simulink model "Fx_observer"  (R2023a)
settings: Solver=ode45  StartTime=0  StopTime=25  FixedStep=0.002  RelTol=1e-3  AbsTol=1e-6
InitFcn:
  | Reff = 0.287;
  | J = 0.8;
libraries: Solver_SF x1
settings Model: ExtModeTrigMode=oneshot  Creator=ywata  LastModifiedBy=USER
settings SolverCC: AutoScaleAbsTol=off  AlgebraicLoopSolver=TrustRegion
settings DataIOCC: SaveFormat=Array  SignalLoggingSaveFormat=ModelDataLogs  ReturnWorkspaceOutputs=off  SignalLoggingName=sigsOut
settings OptimizationCC: BlockReduction=off  BooleanDataType=off  ExpressionDepthLimit=2147483647  LifeSpan=inf
settings DebuggingCC: SaveWithParameterizedLinksMsg=none  UnderspecifiedInitializationDetection=Classic  MergeDetectMultiDrivingBlocksExec=none  SignalResolutionControl=TryResolveAllWithWarning  MultiTaskDSMMsg=warning  MultiTaskCondExecSysMsg=none  FcnCallInpInsideContextMsg=warning  UnconnectedInputMsg=warning  UnconnectedOutputMsg=warning  UnconnectedLineMsg=warning  StateNameClashWarn=warning  SFUnexpectedBacktrackingDiag=warning  SFNoUnconditionalDefaultTransitionDiag=warning  SFExecutionAtInitializationDiag=none  ArithmeticOperatorsInVariantConditions=warning
settings HardwareCC: ProdBitPerPointer=32  ProdBitPerSizeT=32  ProdBitPerPtrDiffT=32  ProdLargestAtomicFloat=None  ProdIntDivRoundTo=Undefined  ProdEndianess=Unspecified  ProdWordSize=32  ProdHWDeviceType=32-bit Generic  TargetUnknown=on
settings ModelReferenceCC: PropagateSignalLabelsOutOfModel=off
settings SFSimCC: SimUseLocalCustomCode=off  CustomCodeUndefinedFunction=UseInterfaceOnly
settings RTWCC: TemplateMakefile=grt_vc.tmf  RTWUseLocalCustomCode=off
settings CodeAppCC: StateflowObjectComments=on
settings GRTTargetCC: TargetFcnLib=ansi_tfl_tmw.mat  TargetLangStandard=C89/C90 (ANSI)  CombineOutputUpdateFcns=off  GRTInterface=on
settings ConfigComp: CovMetricSettings=dw  CovSaveCumulativeToWorkspaceVar=on  CovSaveSingleToWorkspaceVar=on  CovExternalEMLEnable=off

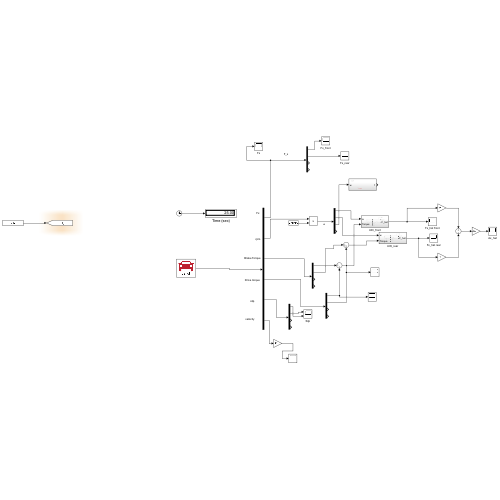
[thumbnail: Simulink's stored preview of the top-level diagram]
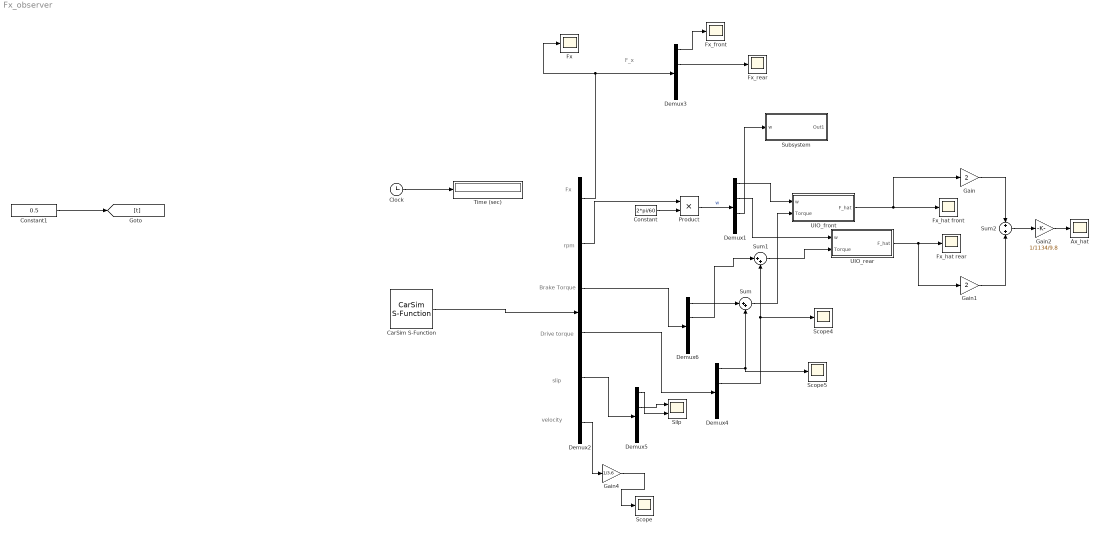
== system Fx_observer ==
  note: velocity
  note: slip
  note: Brake Torque
  note: Fx
  note: Drive torque
  note: rpm
  note: F_x
  Ax_hat : Scope
  CarSim S-Function : Solver_SF/CarSim S-Function  Priority=1  SIMFILE=simfile.sim  Run_RTs=off  vs_state_ind=Run  StopMode_ind=Vehicle Model
  Clock : Clock
  Constant : Constant  Value=2*pi/60
  Constant1 : Constant  Value=0.5
  Demux{1,3..6} (5 alike) : Demux  Outputs=[1 1 1 1]
      settings: DisplayOption=none
  Demux2 : Demux  Outputs=[4 4 4 4 4 1]
      settings: DisplayOption=none
  Fx : Scope
  Fx_front : Scope
  Fx_hat front : Scope
  Fx_hat rear : Scope
  Fx_rear : Scope
  Gain : Gain  Gain=2
  Gain1 : Gain  Gain=2
  Gain2 : Gain  Gain=1/1134/9.8
  Gain4 : Gain  Gain=1/3.6
  Product : Product
  Scope : Scope
  Scope4 : Scope
  Scope5 : Scope
  Silp : Scope  NumInputPorts=2
  Subsystem : Subsystem
  Sum : Sum  Inputs=|++
  Sum1 : Sum  Inputs=|++
  Sum2 : Sum  Inputs=+|+
  Time (sec) : Display
      settings: Format=bank  Decimation=100
  UIO_front : Subsystem
  UIO_rear : Subsystem
  wires:
  Clock/1 -> Time (sec)/1
  Demux2/1 -> Fx/1, Demux3/1
  Demux2/3 -> Demux6/1
  CarSim S-Function/1 -> Demux2/1
  Demux2/2 -> Product/1
  Constant/1 -> Product/2
  Product/1 -> Demux1/1  "w"
  Demux1/2 -> UIO_rear/1(w)
  UIO_rear/1(F_hat) -> Gain1/1, Fx_hat rear/1
  Demux3/1 -> Fx_front/1
  Demux2/4 -> Demux4/1
  Demux2/5 -> Demux5/1
  Demux3/2 -> Fx_rear/1
  Demux4/2 -> Sum1/2, Scope4/1
  Demux1/1 -> UIO_front/1(w)
  UIO_front/1(F_hat) -> Gain/1, Fx_hat front/1
  Demux6/1 -> Sum/1
  Demux4/1 -> Sum/2, Scope5/1
  Sum/1 -> UIO_front/2(Torque)
  Demux6/2 -> Sum1/1
  Sum1/1 -> UIO_rear/2(Torque)
  Gain/1 -> Sum2/1
  Gain1/1 -> Sum2/2
  Sum2/1 -> Gain2/1
  Gain2/1 -> Ax_hat/1
  Demux5/2 -> Silp/1
  Demux2/6 -> Gain4/1
  Gain4/1 -> Scope/1
  Demux5/1 -> Silp/2
  Constant1/1 -> [t]
  Demux1/3 -> Subsystem/1(w)

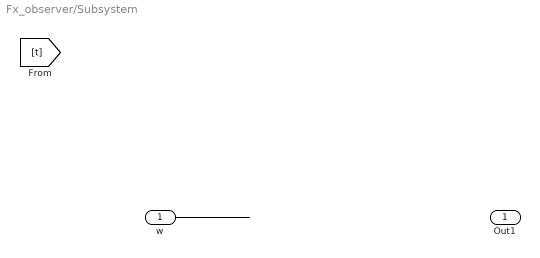
== system Fx_observer/Subsystem ==
  w : Inport
  Out1 : Outport
  wires:
  w/1 -> ?

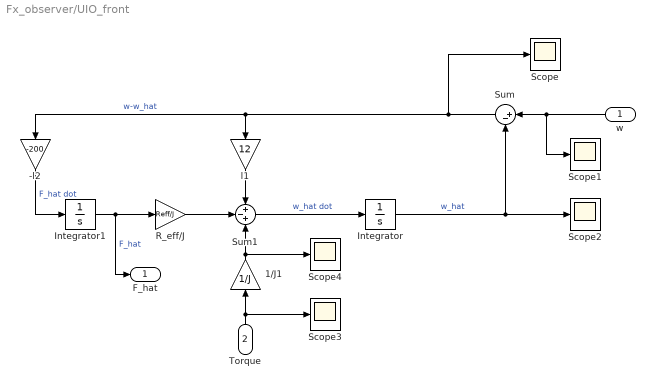
== system Fx_observer/UIO_front ==
  w : Inport
  Torque : Inport  Port=2
  -l2 : Gain  Gain=-200
  1/J1 : Gain  Gain=1/J
  Integrator : Integrator
  Integrator1 : Integrator
  R_eff/J : Gain  Gain=Reff/J
  Scope{,1..4} (5 alike) : Scope
  Sum : Sum  Inputs=|+-
  Sum1 : Sum  Inputs=+-+
  l1 : Gain  Gain=12
  F_hat : Outport
  wires:
  w/1 -> Scope1/1, Sum/1
  Integrator/1 -> Sum/2, Scope2/1  "w_hat"
  Sum1/1 -> Integrator/1  "w_hat dot"
  Sum/1 -> Scope/1, -l2/1, l1/1  "w-w_hat"
  l1/1 -> Sum1/1
  -l2/1 -> Integrator1/1  "F_hat dot"
  Integrator1/1 -> F_hat/1, R_eff/J/1  "F_hat"
  R_eff/J/1 -> Sum1/2
  Torque/1 -> 1/J1/1, Scope3/1
  1/J1/1 -> Sum1/3, Scope4/1

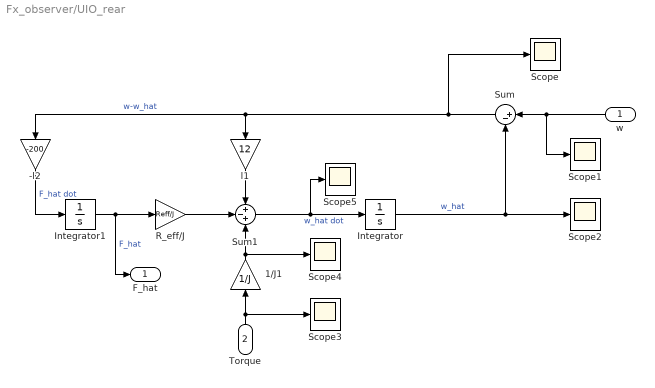
== system Fx_observer/UIO_rear ==
  w : Inport
  Torque : Inport  Port=2
  -l2 : Gain  Gain=-200
  1/J1 : Gain  Gain=1/J
  Integrator : Integrator
  Integrator1 : Integrator
  R_eff/J : Gain  Gain=Reff/J
  Scope{,1..5} (6 alike) : Scope
  Sum : Sum  Inputs=|+-
  Sum1 : Sum  Inputs=+-+
  l1 : Gain  Gain=12
  F_hat : Outport
  wires:
  w/1 -> Scope1/1, Sum/1
  Integrator/1 -> Sum/2, Scope2/1  "w_hat"
  Sum1/1 -> Scope5/1, Integrator/1  "w_hat dot"
  Sum/1 -> Scope/1, -l2/1, l1/1  "w-w_hat"
  l1/1 -> Sum1/1
  -l2/1 -> Integrator1/1  "F_hat dot"
  Integrator1/1 -> F_hat/1, R_eff/J/1  "F_hat"
  R_eff/J/1 -> Sum1/2
  Torque/1 -> 1/J1/1, Scope3/1
  1/J1/1 -> Sum1/3, Scope4/1
